simulink library "INT_CoME_DemCoord"  (R2016b)
settings: Solver=VariableStepAuto  StartTime=0.0  StopTime=10.0  RelTol=1e-3
settings Model: Creator=Administrator  LastModifiedBy=Administrator

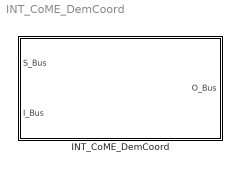
== system INT_CoME_DemCoord ==
  INT_CoME_DemCoord : Subsystem

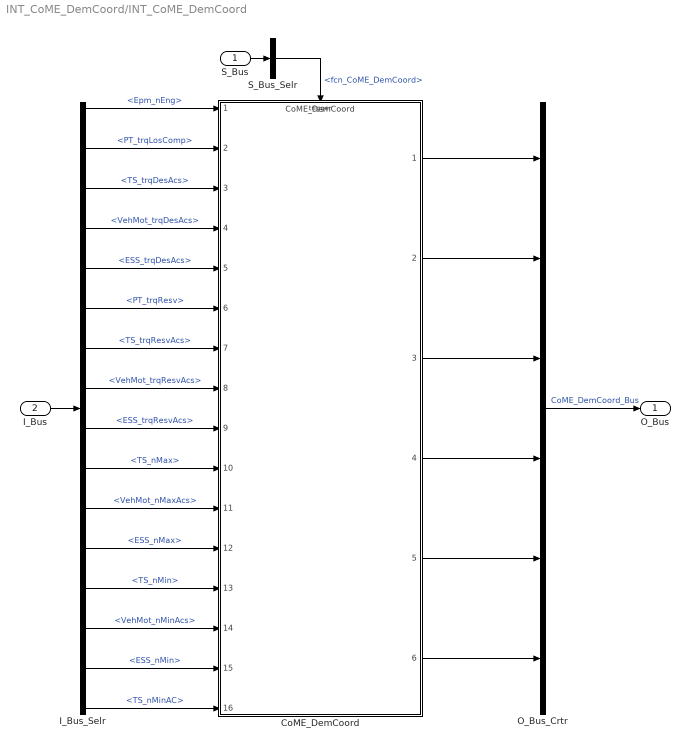
== system INT_CoME_DemCoord/INT_CoME_DemCoord ==
  S_Bus : Inport
  I_Bus : Inport  Port=2
  CoME_DemCoord : ModelReference  ModelNameDialog=CoME_DemCoord  SimulationMode=Normal  ModelReferenceVersion=1.10  TriggerPortName=function  TriggerPortTriggerType=function-call  TriggerPortStatesWhenEnabling=held
  I_Bus_Selr : BusSelector  OutputSignals=Epm_nEng,PT_trqLosComp,TS_trqDesAcs,VehMot_trqDesAcs,ESS_trqDesAcs,PT_trqResv,TS_trqResvAcs,VehMot_trqResvAcs,ESS_trqResvAcs,TS_nMax,VehMot_nMaxAcs,ESS_nMax,TS_nMin,VehMot_nMinAcs,ESS_nMin,TS_nMinAC
  O_Bus_Crtr : BusCreator  Inputs=6
  S_Bus_Selr : BusSelector  OutputSignals=fcn_CoME_DemCoord
  O_Bus : Outport
  wires:
  S_Bus_Selr/1 -> CoME_DemCoord/Trigger  "<fcn_CoME_DemCoord>"
  S_Bus/1 -> S_Bus_Selr/1
  I_Bus/1 -> I_Bus_Selr/1
  I_Bus_Selr/1 -> CoME_DemCoord/1  "<Epm_nEng>"
  I_Bus_Selr/2 -> CoME_DemCoord/2  "<PT_trqLosComp>"
  I_Bus_Selr/3 -> CoME_DemCoord/3  "<TS_trqDesAcs>"
  I_Bus_Selr/4 -> CoME_DemCoord/4  "<VehMot_trqDesAcs>"
  I_Bus_Selr/5 -> CoME_DemCoord/5  "<ESS_trqDesAcs>"
  I_Bus_Selr/6 -> CoME_DemCoord/6  "<PT_trqResv>"
  I_Bus_Selr/7 -> CoME_DemCoord/7  "<TS_trqResvAcs>"
  I_Bus_Selr/8 -> CoME_DemCoord/8  "<VehMot_trqResvAcs>"
  I_Bus_Selr/9 -> CoME_DemCoord/9  "<ESS_trqResvAcs>"
  I_Bus_Selr/10 -> CoME_DemCoord/10  "<TS_nMax>"
  I_Bus_Selr/11 -> CoME_DemCoord/11  "<VehMot_nMaxAcs>"
  I_Bus_Selr/12 -> CoME_DemCoord/12  "<ESS_nMax>"
  I_Bus_Selr/13 -> CoME_DemCoord/13  "<TS_nMin>"
  I_Bus_Selr/14 -> CoME_DemCoord/14  "<VehMot_nMinAcs>"
  I_Bus_Selr/15 -> CoME_DemCoord/15  "<ESS_nMin>"
  I_Bus_Selr/16 -> CoME_DemCoord/16  "<TS_nMinAC>"
  O_Bus_Crtr/1 -> O_Bus/1  "CoME_DemCoord_Bus"
  CoME_DemCoord/1 -> O_Bus_Crtr/1
  CoME_DemCoord/2 -> O_Bus_Crtr/2
  CoME_DemCoord/3 -> O_Bus_Crtr/3
  CoME_DemCoord/4 -> O_Bus_Crtr/4
  CoME_DemCoord/5 -> O_Bus_Crtr/5
  CoME_DemCoord/6 -> O_Bus_Crtr/6
